simulink model "formation"  (R2021b)
settings: Solver=ode15s  StartTime=0.0  StopTime=15  MaxStep=0.01  RelTol=1e-3
undefined symbols (not defined in the file): adj_matrix, delta0_i0, is_0_access, k1, k2, Num, p0_0, q0, v0_0, X, Y, Z
libraries: sm_lib x4, nesl_utility x1
settings Model: PacingRate=1000  Creator=jeff  LastModifiedBy=jeff
settings SolverCC: ZeroCrossAlgorithm=Adaptive  SolverResetMethod=Robust

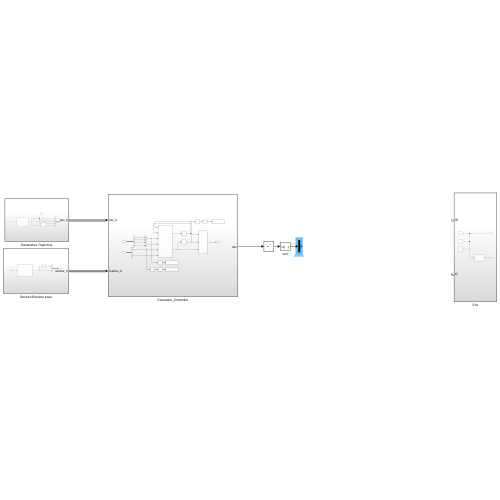
[thumbnail: Simulink's stored preview of the top-level diagram]
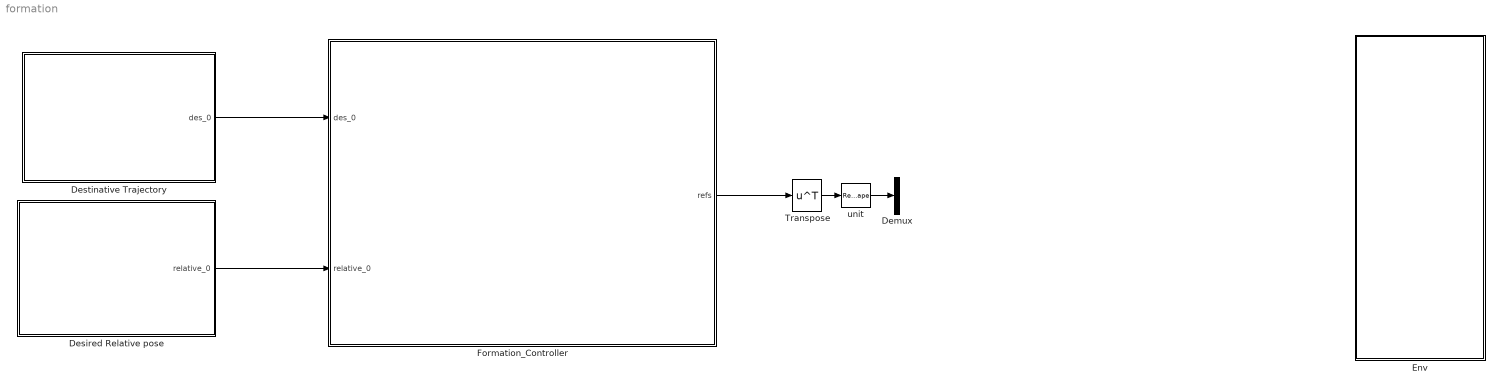
== system formation ==
  Demux : Demux  Outputs=1
  Desired Relative pose : Subsystem
  Destinative Trajectory : Subsystem
  Env : Subsystem
  Formation_Controller : Subsystem
  Transpose : Math  Operator=transpose  SaturateOnIntegerOverflow=on
  unit : Reshape
  wires:
  Destinative Trajectory/1(des_0) -> Formation_Controller/1(des_0)
  Desired Relative pose/1(relative_0) -> Formation_Controller/2(relative_0)
  unit/1 -> Demux/1
  Formation_Controller/1(refs) -> Transpose/1
  Transpose/1 -> unit/1

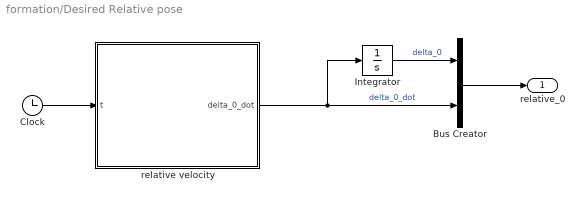
== system formation/Desired Relative pose ==
  Bus Creator : BusCreator  Inputs=2
  Clock : Clock
  Integrator : Integrator  InitialCondition=delta0_i0
  relative velocity : MATLAB Function  TreatAsAtomicUnit=on
  relative_0 : Outport
  wires:
  Clock/1 -> relative velocity/1(t)
  relative velocity/1(delta_0_dot) -> Bus Creator/2, Integrator/1  "delta_0_dot"
  Bus Creator/1 -> relative_0/1
  Integrator/1 -> Bus Creator/1  "delta_0"

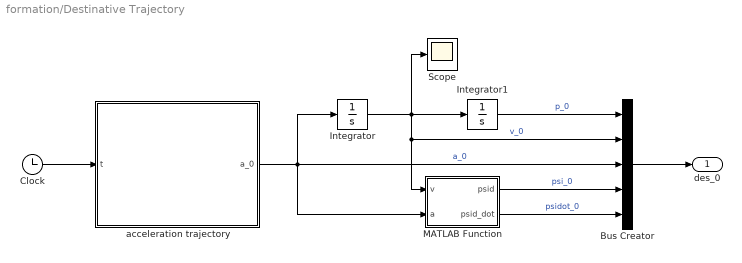
== system formation/Destinative Trajectory ==
  Bus Creator : BusCreator  Inputs=5
  Clock : Clock
  Integrator : Integrator  InitialCondition=v0_0
  Integrator1 : Integrator  InitialCondition=p0_0
  MATLAB Function : MATLAB Function  TreatAsAtomicUnit=on
  Scope : Scope
  acceleration trajectory : MATLAB Function  TreatAsAtomicUnit=on
  des_0 : Outport
  wires:
  Clock/1 -> acceleration trajectory/1(t)
  acceleration trajectory/1(a_0) -> MATLAB Function/2(a), Integrator/1, Bus Creator/3  "a_0"
  Integrator/1 -> Scope/1, Integrator1/1, Bus Creator/2, MATLAB Function/1(v)  "v_0"
  Integrator1/1 -> Bus Creator/1  "p_0"
  Bus Creator/1 -> des_0/1
  MATLAB Function/2(psid_dot) -> Bus Creator/5  "psidot_0"
  MATLAB Function/1(psid) -> Bus Creator/4  "psi_0"

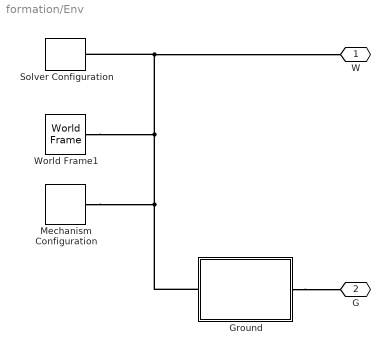
== system formation/Env ==
  Ground : Subsystem
  Mechanism Configuration : sm_lib/Utilities/Mechanism Configuration  UniformGravity=Constant  GravityVector=[0 0 -9.80665]  GravityUnits=m/s^2  LinearizationDelta=0.001  JointModeTransitionNonlinearIterations=2
  Solver Configuration : nesl_utility/Solver Configuration  PhysicalDomain=network_engine_domain  SubClassName=solver  LeftPortType=input  RightPortType=generic  Tones=[]  Harmonics=[]  SimulateNoise=off  Profile=off  UseLocalSampling=off  EnableSwitchedLinearOptims=on  FrequencyDomain=off  UseCCode=off  RelTol=0.001  AbsTol=1e-06  MinStep=1e-09  ToWorkspace=off  RevertToSquareIcSolve=off  NumHomotopyIterations=100  PhasorMode=off  PhasorModeNumHarmonics=1  DoDC=off  ResidualTolerance=1e-09  UseLocalSolver=off  LocalSolverChoice=NE_BACKWARD_EULER_ADVANCER  LocalSolverSampleTime=0.001  DoFixedCost=off  MaxNonlinIter=3  MaxModeIter=2  ComputeImpulses=off  ImpulseIterations=2  LinearAlgebra=Sparse  EquationFormulation=NE_TIME_EF  DelaysMemoryBudget=1024  AutomaticFiltering=on  FilteringTimeConstant=0.001  PartitionStorageMethod=AS_NEEDED  PartitionMemoryBudget=1024  PartitionMethod=FAST
      settings: SourceProductBaseCode=PW,SS
  World Frame1 : sm_lib/Frames and Transforms/World Frame
  W : PMIOPort  Side=Left
  G : PMIOPort  Port=2  Side=Left
  connections:
  Ground/RConn1 -- G/RConn1
  Ground/LConn1 -- Mechanism Configuration/RConn1 -- World Frame1/RConn1 -- Solver Configuration/RConn1 -- W/RConn1

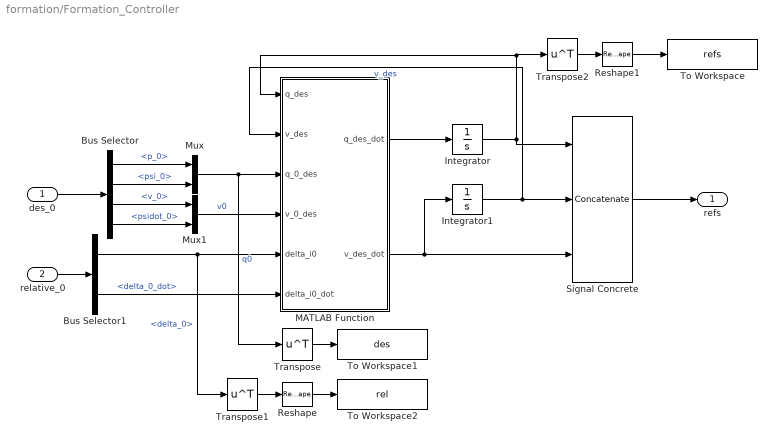
== system formation/Formation_Controller ==
  des_0 : Inport
  relative_0 : Inport  Port=2
  Bus Selector : BusSelector  OutputSignals=p_0,psi_0,v_0,psidot_0
  Bus Selector1 : BusSelector  OutputSignals=delta_0,delta_0_dot
  Integrator : Integrator  InitialCondition=q0
  Integrator1 : Integrator  InitialCondition=zeros(Num,4)
  MATLAB Function : MATLAB Function  TreatAsAtomicUnit=on
  Mux : Mux  Inputs=2
  Mux1 : Mux  Inputs=2
  Reshape : Reshape
  Reshape1 : Reshape
  Signal Concrete : Concatenate  NumInputs=3  Mode=Multidimensional array  ConcatenateDimension=2
  To Workspace : ToWorkspace  VariableName=refs  SampleTime=-1
      settings: Save2DSignal=2-D array (concatenate along first dimension)
  To Workspace1 : ToWorkspace  VariableName=des  SampleTime=-1
      settings: Save2DSignal=2-D array (concatenate along first dimension)
  To Workspace2 : ToWorkspace  VariableName=rel  SampleTime=-1
      settings: Save2DSignal=2-D array (concatenate along first dimension)
  Transpose : Math  Operator=transpose  SaturateOnIntegerOverflow=on
  Transpose1 : Math  Operator=transpose  SaturateOnIntegerOverflow=on
  Transpose2 : Math  Operator=transpose  SaturateOnIntegerOverflow=on
  refs : Outport
  wires:
  des_0/1 -> Bus Selector/1
  Bus Selector/1 -> Mux/1  "<p_0>"
  Bus Selector/2 -> Mux/2  "<psi_0>"
  Mux/1 -> MATLAB Function/3(q_0_des), Transpose/1  "q0"
  Bus Selector/4 -> Mux1/2  "<psidot_0>"
  Bus Selector/3 -> Mux1/1  "<v_0>"
  Mux1/1 -> MATLAB Function/4(v_0_des)  "v0"
  MATLAB Function/1(q_des_dot) -> Integrator/1
  MATLAB Function/2(v_des_dot) -> Integrator1/1, Signal Concrete/3
  Integrator/1 -> MATLAB Function/1(q_des), Transpose2/1, Signal Concrete/1
  Integrator1/1 -> MATLAB Function/2(v_des), Signal Concrete/2  "v_des"
  relative_0/1 -> Bus Selector1/1
  Bus Selector1/1 -> Transpose1/1, MATLAB Function/5(delta_i0)  "<delta_0>"
  Bus Selector1/2 -> MATLAB Function/6(delta_i0_dot)  "<delta_0_dot>"
  Signal Concrete/1 -> refs/1
  Transpose/1 -> To Workspace1/1
  Reshape/1 -> To Workspace2/1
  Reshape1/1 -> To Workspace/1
  Transpose1/1 -> Reshape/1
  Transpose2/1 -> Reshape1/1

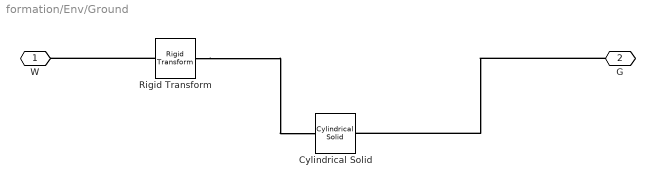
== system formation/Env/Ground ==
  Cylindrical Solid : sm_lib/Body Elements/Cylindrical Solid  GraphicAmbientColor=[0.15 0.15 0.15 1.0]  BasedOnType=Mass  CenterOfMass=[0 0 0]  CenterOfMassUnits=m  GraphicDiffuseColor=[0.8 1.0 0.8]  CylinderLength=10  CylinderLengthUnits=mm  CylinderRadius=4  CylinderRadiusUnits=m  Density=1000  DensityUnits=kg/m^3  DoExposeReferenceFrame=off  GraphicEmissiveColor=[0.0 0.0 0.0 1.0]  ExportEntireGeometry=on  SerializedFrames=<Frames><Frame><Id>Frame1</Id><Value><Name>F1</Name><Origin><Source>GeometricFeature</Source><FeatureName>top surface</FeatureName></Origin><PrimaryAxis><DefinedDirection>+Z</DefinedDirection><Source>ReferenceFrame</Source><SourceDirection>+Z</SourceDirection><FeatureName></FeatureName></PrimaryAxis><SecondaryAxis><DefinedDirection>+X</DefinedDirection><Source>ReferenceFrame</Source><SourceDirection>+X</SourceDirection><FeatureName></FeatureName></SecondaryAxis></Value></Frame></Frames>  MarkerShape=Sphere  MarkerSize=10  GraphicType=FromGeometry  InertiaType=Custom  Mass=0  MassUnits=kg  MomentsOfInertia=[1 1 1]  MomentsOfInertiaUnits=kg*m^2  GraphicOpacity=1.0  ProductsOfInertia=[0 0 0]  ProductsOfInertiaUnits=kg*m^2  GraphicShininess=75  GraphicSpecularColor=[0.5 0.5 0.5 1.0]  GraphicVisPropType=SimpleVisualProperties
  Rigid Transform : sm_lib/Frames and Transforms/Rigid Transform  TranslationMethod=StandardAxis  TranslationStandardOffset=6  TranslationLengthUnit=cm  TranslationStandardAxis=-Z  TranslationCartesianOffset=[0 0 0]  TranslationROffset=0  TranslationROffsetUnits=m  TranslationZOffset=0  TranslationZOffsetUnits=m  TranslationThetaOffset=0  TranslationThetaOffsetUnits=deg  RotationMethod=None  RotationAngleUnits=deg  RotationStandardAxis=+Z  RotationAngle=0.0  RotationArbitraryAxis=[0 0 1]  FollAlignAxisA=+X  BaseAlignAxisA=+Y  FollAlignAxisB=+Y  BaseAlignAxisB=+Z  RotationSequenceAxes=FollowerAxes  RotationSequence=XYX  RotationSequenceAngles=[0 0 0]  RotationSequenceAnglesUnits=deg  RotationMatrix=[1 0 0; 0 1 0; 0 0 1]
  W : PMIOPort  Side=Left
  G : PMIOPort  Port=2  Side=Right
  connections:
  G/RConn1 -- Cylindrical Solid/RConn1
  Rigid Transform/LConn1 -- W/RConn1
  Rigid Transform/RConn1 -- Cylindrical Solid/LConn1

== matlab function formation/Destinative Trajectory/MATLAB Function ==
  data: v input; psid output; a input; psid_dot output
function [psid, psid_dot] = fcn(v,a)
% x_dot = v(1);
% y_dot = v(2);
% x_ddot = a(1);
% y_ddot = a(2);
% psid = atan2(y_dot,x_dot);
% if x_dot<0 && x_dot>-1e-2
%     psid=atan2(y_dot,-x_dot);
% end
% if x_dot==0 && y_dot==0
%     psid_dot = 0;
% else
%     psid_dot = (-x_ddot*y_dot-y_ddot*x_dot)/(x_dot^2+y_dot^2);
% end
psid = 0;
psid_dot = 0;

== matlab function formation/Destinative Trajectory/acceleration trajectory ==
  data: t input; a_0 output
function a_0 = fcn_a_0(t)
a_0 = f_a_0(t);

== matlab function formation/Formation_Controller/MATLAB Function ==
  data: q_des input; v_des input; q_0_des input; v_0_des input; delta_i0 input; delta_i0_dot input; q_des_dot output size=[Num,4]; Num parameter; v_des_dot output size=[Num,4]; k1 parameter; k2 parameter; adj_matrix parameter; is_0_access parameter
function [q_des_dot, v_des_dot] = fcn(q_des, v_des, q_0_des, v_0_des, delta_i0, delta_i0_dot, Num, k1, k2, adj_matrix, is_0_access)
q_des_dot=zeros(Num,4);
v_des_dot=zeros(Num,4);

for i=1:Num
    q_des_dot(i,:) = v_des(i,:) - k1*is_0_access(i)*(qsubtract(q_des(i,:),q_0_des')-delta_i0(i,:));
    for j=1:Num
        q_des_dot(i,:) = q_des_dot(i,:) - k1*adj_matrix(i,j)*(qsubtract(q_des(i,:),q_des(j,:))-(delta_i0(i,:)-delta_i0(j,:)));
    end
    v_des_dot(i,:) = -k2*is_0_access(i)*(v_des(i,:)-v_0_des'-delta_i0_dot(i,:));
    for j=1:Num
        v_des_dot(i,:) = v_des_dot(i,:)-k2*adj_matrix(i,j)*(v_des(i,:)-v_des(j,:)-(delta_i0_dot(i,:)-delta_i0_dot(j,:)));
    end
end

function Deltaq = qsubtract(q1,q2)
Deltaq = q1 - q2;
if Deltaq(4) > pi
    Deltaq(4) = Deltaq(4) - 2*pi;
elseif Deltaq(4) < -pi
    Deltaq(4) = Deltaq(4) + 2*pi;
end

== matlab function formation/Desired Relative pose/relative velocity ==
  data: t input; delta_0_dot output size=[Num, 4]
function delta_0_dot = rel_vel(t)
delta_0_dot = rel_v(t);
